simulink model "SolarCellModelRepFinal"  (R2016b)
settings: Solver=VariableStepAuto  StartTime=0.0  StopTime=10.0  RelTol=1e-3
undefined symbols (not defined in the file): K, N, q
libraries: simulink x5
settings Model: Creator=hp  LastModifiedBy=hp

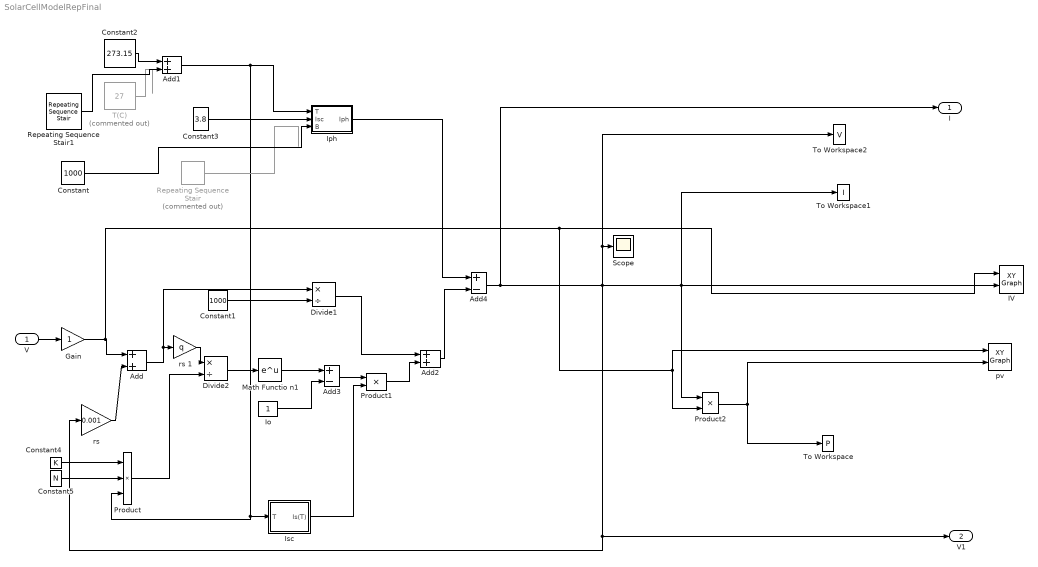
== system SolarCellModelRepFinal ==
  V : Inport
  Add : Sum
  Add1 : Sum
  Add2 : Sum
  Add3 : Sum  Inputs=+-
  Add4 : Sum  Inputs=+-
  Constant : Constant  Value=1000
  Constant1 : Constant  Value=1000
  Constant2 : Constant  Value=273.15
  Constant3 : Constant  Value=3.8
  Constant4 : Constant  Value=K
  Constant5 : Constant  Value=N
  Divide1 : Product  Inputs=*/
  Divide2 : Product  Inputs=*/
  Gain : Gain
  "IV " : simulink/Sinks/XY Graph  xmin=0  xmax=0.7  ymin=0  ymax=30  st=-1
  Io : Constant
  Iph : Subsystem
  Isc : Subsystem
      mask init:
      | q = 1.6e-19;
      | T = 300.15;
      | Tnom = 300.15;
      | K = 1.38e-23;
      | N = 1.5;
      | vt = T*K/q;
      | Is =1e-9;
      | Eg = 1.12;
      | 4
  Math Functio n1 : Math  SaturateOnIntegerOverflow=on
  Product : Product  Inputs=3
  Product1 : Product
  Product2 : Product
  Repeating Sequence Stair : simulink/Sources/Repeating Sequence Stair  Commented=on  OutValues=[1000 800 600 400]  tsamp=1  OutMin=[]  OutMax=[]  OutDataTypeStr=double  OutputDataTypeScalingMode=double  OutDataType=fixdt(0,8)  ConRadixGroup=Best Precision: Vector-wise  OutScaling=2^-12
  Repeating Sequence Stair1 : simulink/Sources/Repeating Sequence Stair  OutValues=[25 30 40 50]  tsamp=1  OutMin=[]  OutMax=[]  OutDataTypeStr=double  OutputDataTypeScalingMode=double  OutDataType=fixdt(0,8)  ConRadixGroup=Best Precision: Vector-wise  OutScaling=2^-12
  Scope : Scope
  T(C) : Constant  Commented=on  Value=27
  To Workspace : ToWorkspace  VariableName=P  SaveFormat=Timeseries  SampleTime=-1
  To Workspace1 : ToWorkspace  VariableName=I  SaveFormat=Timeseries  SampleTime=-1
  To Workspace2 : ToWorkspace  VariableName=V  SaveFormat=Timeseries  SampleTime=-1
  pv : simulink/Sinks/XY Graph  xmin=0  xmax=0.7  ymin=0  ymax=20  st=-1
  "rs " : Gain  Gain=0.001
  rs 1 : Gain  Gain=q
  I : Outport
  V1 : Outport  Port=2
  wires:
  Math Functio n1/1 -> Add3/1
  Product1/1 -> Add2/2
  Gain/1 -> "IV "/1, pv/1, Product2/2, Add/1
  Divide2/1 -> Math Functio n1/1
  "rs "/1 -> Add/2
  Io/1 -> Add3/2
  Add3/1 -> Product1/1
  Add2/1 -> Add4/2
  V/1 -> Gain/1
  Add4/1 -> I/1, To Workspace2/1, Scope/1, To Workspace1/1, "IV "/2, Product2/1, "rs "/1, V1/1
  Add/1 -> rs 1/1, Divide1/1
  Constant1/1 -> Divide1/2
  Divide1/1 -> Add2/1
  Add1/1 -> Product/3, Isc/1(T), Iph/1(T)
  Isc/1(Is(T)) -> Product1/2
  Iph/1(Iph) -> Add4/1
  Product/1 -> Divide2/2
  Constant4/1 -> Product/1
  Constant5/1 -> Product/2
  Constant3/1 -> Iph/2(Isc)
  Repeating Sequence Stair/1 -> ?
  Product2/1 -> pv/2, To Workspace/1
  rs 1/1 -> Divide2/1
  Constant2/1 -> Add1/1
  T(C)/1 -> ?
  Constant/1 -> Iph/3("B ")
  Repeating Sequence Stair1/1 -> Add1/2

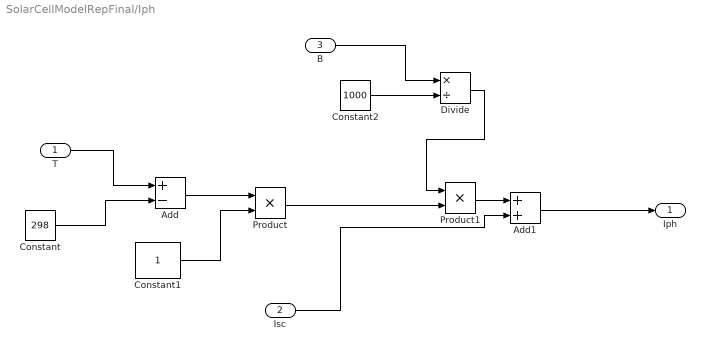
== system SolarCellModelRepFinal/Iph ==
  T : Inport
  Isc : Inport  Port=2
  "B " : Inport  Port=3
  Add : Sum  Inputs=+-
  Add1 : Sum
  Constant : Constant  Value=298
  Constant1 : Constant
  Constant2 : Constant  Value=1000
  Divide : Product  Inputs=*/
  Product : Product
  Product1 : Product
  Iph : Outport
  wires:
  Constant/1 -> Add/2
  T/1 -> Add/1
  Add/1 -> Product/1
  Constant1/1 -> Product/2
  Product/1 -> Product1/2
  Isc/1 -> Add1/2
  Add1/1 -> Iph/1
  Divide/1 -> Product1/1
  Constant2/1 -> Divide/2
  "B "/1 -> Divide/1
  Product1/1 -> Add1/1

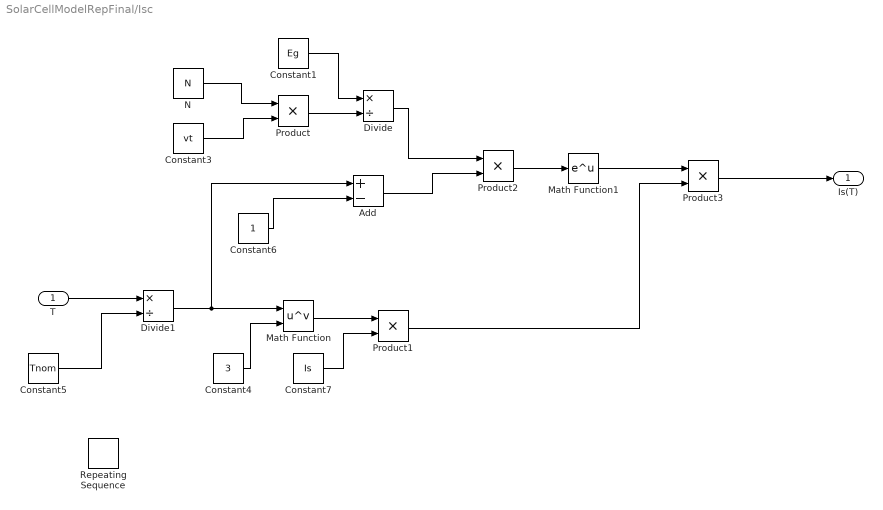
== system SolarCellModelRepFinal/Isc ==
  T : Inport
  Add : Sum  Inputs=+-
  Constant1 : Constant  Value=Eg
  Constant3 : Constant  Value=vt
  Constant4 : Constant  Value=3
  Constant5 : Constant  Value=Tnom
  Constant6 : Constant
  Constant7 : Constant  Value=Is
  Divide : Product  Inputs=*/
  Divide1 : Product  Inputs=*/
  Math Function : Math  Operator=pow  SaturateOnIntegerOverflow=on
  Math Function1 : Math  SaturateOnIntegerOverflow=on
  N : Constant  Value=N
  Product{,1..3} (4 alike) : Product
  Repeating Sequence : simulink/Sources/Repeating Sequence  rep_seq_t=[0 1 2]  rep_seq_y=[-0.1 0.6 -0.1]
  Is(T) : Outport
  wires:
  Constant1/1 -> Divide/1
  Product/1 -> Divide/2
  N/1 -> Product/1
  Constant3/1 -> Product/2
  Constant6/1 -> Add/2
  Divide1/1 -> Math Function/1, Add/1
  T/1 -> Divide1/1
  Constant5/1 -> Divide1/2
  Constant4/1 -> Math Function/2
  Math Function/1 -> Product1/1
  Constant7/1 -> Product1/2
  Divide/1 -> Product2/1
  Add/1 -> Product2/2
  Product2/1 -> Math Function1/1
  Math Function1/1 -> Product3/1
  Product1/1 -> Product3/2
  Product3/1 -> Is(T)/1
